simulink model "Jumper_Elastica"  (R2017b)
settings: Solver=ode15s  StartTime=0.0  StopTime=2  MaxStep=1e-2  RelTol=1e-3  EnableMultiTasking=on
InitFcn:
  | Variable_initialisation
values from neighbouring files (symbols this model uses):
  ArmatureResistance = 3.89    [Variable_initialisation.m]    (also in Variable_initialisation_shortleg.m; Variable_inizializzazione.m)
  ArmLength = 1.5    [Variable_initialisation.m]    (also in Variable_initialisation_shortleg.m; Variable_inizializzazione.m)
  ArmWidth = 0.1    [Variable_initialisation.m]    (also in Variable_initialisation_shortleg.m; Variable_inizializzazione.m)
  BaseX = Base*cos(BaseAngle)    [Variable_initialisation.m]    (also in Variable_initialisation_shortleg.m; Variable_inizializzazione.m; fourbar_initialisation.m)
  BaseY = Base*sin(BaseAngle)    [Variable_initialisation.m]    (also in Variable_initialisation_shortleg.m; Variable_inizializzazione.m; fourbar_initialisation.m)
  BodyMass = 1.0    (= 1)    [Variable_initialisation.m]    (also in Variable_initialisation_shortleg.m; Variable_inizializzazione.m = 1.4)
  FrontThigh = 30*Scale    (= 60)    [Variable_initialisation.m]    (also in Variable_initialisation_shortleg.m; Variable_inizializzazione.m; fourbar_initialisation.m = 45)
  GearRatio = 30    [Variable_initialisation.m]    (also in Variable_initialisation_shortleg.m; Variable_inizializzazione.m)
  Gravity = 9.81    [Variable_initialisation.m]    (also in Variable_initialisation_shortleg.m; Variable_inizializzazione.m)
  HardStop = 170    [Variable_initialisation.m]    (also in Variable_initialisation_shortleg.m; Variable_inizializzazione.m)
  InitialAngle = -113    [Variable_initialisation.m]    (also in Variable_initialisation_shortleg.m; Variable_inizializzazione.m)
  JumpingLegAttachPoint = -0.05    [Variable_initialisation.m]    (also in Variable_initialisation_shortleg.m = 0.05; Variable_inizializzazione.m)
  JumpingLegLength = 1.2    [Variable_initialisation.m]    (also in Variable_initialisation_shortleg.m = 0.9; Variable_inizializzazione.m = 0.8)
  JumpingLegMass = 0.3    [Variable_initialisation.m]    (also in Variable_initialisation_shortleg.m; Variable_inizializzazione.m = 0.5)
  JumpingLegStartAngle = rad2deg(asin(LandingLegHeight/JumpingLegCompressedLength))    [Variable_initialisation.m]    (also in Variable_initialisation_shortleg.m; Variable_inizializzazione.m)
  Knee = 5*Scale    (= 10)    [Variable_initialisation.m]    (also in Variable_initialisation_shortleg.m; Variable_inizializzazione.m; fourbar_initialisation.m)
  LandingLegHeight = 0.5    [Variable_initialisation.m]    (also in Variable_initialisation_shortleg.m; Variable_inizializzazione.m)
  LandingLegMass = 0.1    [Variable_initialisation.m]    (also in Variable_initialisation_shortleg.m; Variable_inizializzazione.m)
  MotorFreeSpeed = 2027    [Variable_initialisation.m]    (also in Variable_initialisation_shortleg.m; Variable_inizializzazione.m)
  MotorStallTorque = 2.32    [Variable_initialisation.m]    (also in Variable_initialisation_shortleg.m; Variable_inizializzazione.m)
  MotorVoltage = 16    [Variable_initialisation.m]    (also in Variable_initialisation_shortleg.m; Variable_inizializzazione.m)
  RearThigh = 29.5*Scale    (= 59)    [Variable_initialisation.m]    (also in Variable_initialisation_shortleg.m; Variable_inizializzazione.m; fourbar_initialisation.m = 43.5)
  SEA_Spring = 1e6    (= 1000000)    [Variable_initialisation.m]    (also in Variable_initialisation_shortleg.m; Variable_inizializzazione.m)
  Shin = 30*Scale    (= 60)    [Variable_initialisation.m]    (also in Variable_initialisation_shortleg.m; Variable_inizializzazione.m; fourbar_initialisation.m = 45)
undefined symbols (not defined in the file or in its folder): Beam, beam_wall, beam_width, Extr_Data_Box, magnitude, X, Y, Z
libraries: sm_lib x67, nesl_utility x25, fl_lib x21, simulink x8, Contact_Forces_Lib x7, sm_flex_body_lib x5, powerlib_meascontrol x2, mblibv1 x1, elec_lib x1
(part 1 of 3)
settings Model: Creator=rjs08  LastModifiedBy=rjs08
settings DataIOCC: LimitDataPoints=on
settings OptimizationCC: LifeSpan=inf
settings DebuggingCC: AllowSymbolicDim=off  SFUnexpectedBacktrackingDiag=warning  SFNoUnconditionalDefaultTransitionDiag=warning  SFExecutionAtInitializationDiag=none
settings CodeAppCC: StateflowObjectComments=on
settings GRTTargetCC: TargetLangStandard=C89/C90 (ANSI)  GeneratePreprocessorConditionals=Disable all
settings ConfigComp: CovMetricSettings=dw  CovHtmlReporting=on  CovSaveCumulativeToWorkspaceVar=on  CovSaveSingleToWorkspaceVar=on  CovExternalEMLEnable=off  CovSFcnEnable=off
settings SimscapeCC: SimscapeNominalValues="[{\"value\":\"10\",\"unit\":\"V\"},{\"value\":\"1\",\"unit\":\"A\"},{\"value\":\"10\",\"unit\":\"N*m\"},{\"value\":\"10\",\"unit\":\"bar\"},{\"value\":\"100\",\"unit\":\"kJ/kg\"},{\"value\":\"1\",\"unit\":\"kW\"},{\"value\":\"300\",\"unit\":\"K\"},{\"value\":\"100\",\"unit\":\"cm^3/s\"},{\"value\":\"1\",\"unit\":\"kN\"},{\"value\":\"1\",\"unit\":\"g/cm^3\"},{\"value\":\"1\",\"unit\":\"l\"},{\"value\":\"1\",\"unit\":\"cm^2\"},{\"value\":\"60\",\"unit\":\"Hz\"}]"  SimscapeLogType=all  SimscapeLogDataHistory=10000
settings ConfigurationSet: Description=SimMechanics 2G
settings DiagnosticsConfigSet: SimMechanicsRigidlyBoundBlock=none

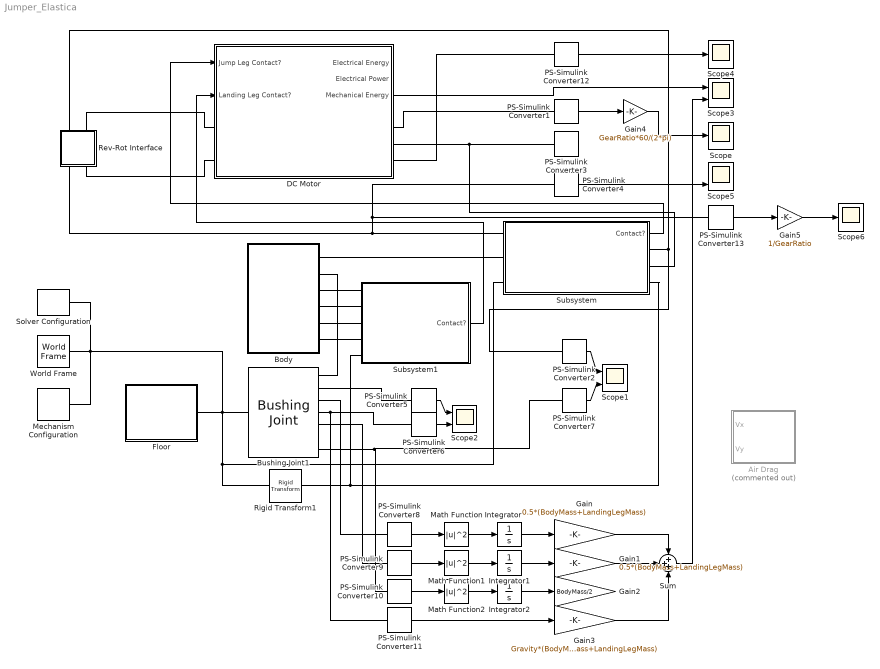
== system Jumper_Elastica ==
  Air Drag : Subsystem  Commented=on  mask(Air friction model){Cd=0}
      mask prompts: Cd "Drag Coefficient"
      mask help: Models aerodynamic drag. The drag coefficient Cd is a mask block parameter. Cd = 0 corresponds to zero drag. Cd = 2 corresponds to a sphere.
      mask init:
      | 0;
      mask Help: Enter aerodynamic drag coefficient Cd.  The block generates a three-vector of air friction as a function of 2D input velocity.
  Body : Subsystem  mask{L=ArmLength, L3=JumpingLegAttachPoint, W=ArmWidth, H=ArmWidth/2, M=BodyMass, LegH=LandingLegHeight, LegM=LandingLegMass, LegL=LandingLegHeight, rgb=[0 0 0]}
      mask prompts: L "Arm Length (m)"; L3 "Motor Mount Point (m)"; W "Arm Width (m)"; H "Body Thickness (m)"; M "Body Mass (kg)"; LegH "Leg Height (m)"; LegM "Leg Mass (kg)"; LegL "Leg Foot Length"; rgb "Color [R G B]"
  Bushing Joint1 : sm_lib/Joints/Bushing Joint  SenseConstraintForce=off  SenseConstraintForceX=off  SenseConstraintForceY=off  SenseConstraintForceZ=off  SenseConstraintTorque=off  SenseConstraintTorqueX=off  SenseConstraintTorqueY=off  SenseConstraintTorqueZ=off  SenseTotalForce=off  SenseTotalForceX=off  SenseTotalForceY=off  SenseTotalForceZ=off  SenseTotalTorque=off  SenseTotalTorqueX=off  SenseTotalTorqueY=off  SenseTotalTorqueZ=off  CompositeWrenchDir=FollowerOnBase  CompositeWrenchFrame=BaseFrame  PxEquilibriumPosition=0  PxEquilibriumPositionUnits=m  PxSpringStiffness=0  PxSpringStiffnessUnits=N/m  PxDampingCoefficient=0  PxDampingCoefficientUnits=N/(m/s)  PxTorqueActuationMode=NoTorque  PxMotionActuationMode=ComputedMotion  PxSensePosition=on  PxSenseVelocity=on  PxSenseAcceleration=off  PxSenseTorqueForce=off  PxPositionTargetSpecify=on  PxPositionTargetPriority=High  PxPositionTargetValue=0  PxPositionTargetValueUnits=m  PxVelocityTargetSpecify=off  PxVelocityTargetPriority=High  PxVelocityTargetValue=0  PxVelocityTargetValueUnits=m/s  PyEquilibriumPosition=0  PyEquilibriumPositionUnits=m  PySpringStiffness=0  PySpringStiffnessUnits=N/m  PyDampingCoefficient=0  PyDampingCoefficientUnits=N/(m/s)  PyTorqueActuationMode=NoTorque  PyMotionActuationMode=ComputedMotion  PySensePosition=on  PySenseVelocity=on  PySenseAcceleration=off  PySenseTorqueForce=off  PyPositionTargetSpecify=on  PyPositionTargetPriority=High  PyPositionTargetValue=0.05  PyPositionTargetValueUnits=m  PyVelocityTargetSpecify=off  PyVelocityTargetPriority=High  PyVelocityTargetValue=0  PyVelocityTargetValueUnits=m/s  PzEquilibriumPosition=0  PzEquilibriumPositionUnits=m  PzSpringStiffness=0  PzSpringStiffnessUnits=N/m  PzDampingCoefficient=0  PzDampingCoefficientUnits=N/(m/s)  PzTorqueActuationMode=NoTorque  PzMotionActuationMode=ComputedMotion  PzSensePosition=off  PzSenseVelocity=off  PzSenseAcceleration=off  PzSenseTorqueForce=off  PzPositionTargetSpecify=on  PzPositionTargetPriority=High  PzPositionTargetValue=0  PzPositionTargetValueUnits=m  PzVelocityTargetSpecify=off  PzVelocityTargetPriority=High  PzVelocityTargetValue=0  PzVelocityTargetValueUnits=m/s  RxEquilibriumPosition=0  RxEquilibriumPositionUnits=deg  RxSpringStiffness=0  RxSpringStiffnessUnits=N*m/deg  RxDampingCoefficient=0  RxDampingCoefficientUnits=N*m/(deg/s)  RxTorqueActuationMode=NoTorque  RxMotionActuationMode=ComputedMotion  RxSensePosition=off  RxSenseVelocity=off  RxSenseAcceleration=off  RxSenseTorqueForce=off  RxPositionTargetSpecify=on  RxPositionTargetPriority=High  RxPositionTargetValue=0  RxPositionTargetValueUnits=deg  RxVelocityTargetSpecify=off  RxVelocityTargetPriority=High  RxVelocityTargetValue=0  RxVelocityTargetValueUnits=deg/s  RyEquilibriumPosition=0  RyEquilibriumPositionUnits=deg  RySpringStiffness=0  RySpringStiffnessUnits=N*m/deg  RyDampingCoefficient=0  RyDampingCoefficientUnits=N*m/(deg/s)  RyTorqueActuationMode=NoTorque  RyMotionActuationMode=ComputedMotion  RySensePosition=off  RySenseVelocity=off  RySenseAcceleration=off  RySenseTorqueForce=off  RyPositionTargetSpecify=on  RyPositionTargetPriority=High  RyPositionTargetValue=0  RyPositionTargetValueUnits=deg  RyVelocityTargetSpecify=off  RyVelocityTargetPriority=High  RyVelocityTargetValue=0  RyVelocityTargetValueUnits=deg/s  RzEquilibriumPosition=0  RzEquilibriumPositionUnits=deg  RzSpringStiffness=0  RzSpringStiffnessUnits=N*m/deg  RzDampingCoefficient=0  RzDampingCoefficientUnits=N*m/(deg/s)  RzTorqueActuationMode=NoTorque  RzMotionActuationMode=ComputedMotion  RzSensePosition=on  RzSenseVelocity=on  RzSenseAcceleration=off  RzSenseTorqueForce=off  RzPositionTargetSpecify=on  RzPositionTargetPriority=High  RzPositionTargetValue=0  RzPositionTargetValueUnits=deg  RzVelocityTargetSpecify=off  RzVelocityTargetPriority=High  RzVelocityTargetValue=0  RzVelocityTargetValueUnits=deg/s
      settings: SourceProductName=Simscape Multibody
  DC Motor : Subsystem  mask{Stall_Torque=MotorStallTorque, Free_Speed=MotorFreeSpeed, Armature_Resistance=ArmatureResistance, Reverse_Point=0.3, Gear_Ratio=GearRatio, Motor_Voltage=MotorVoltage, SEA_Spring=SEA_Spring}
      mask prompts: Stall_Torque "Motor Stall Torque (Nm)"; Free_Speed "Motor Free Speed (rpm)"; Armature_Resistance "Motor Armature Resistance (ohm)"; Reverse_Point "Reverse Point (ignore)"; Gear_Ratio "Gear Reduction Ratio"; Motor_Voltage "Motor Voltage (V)"; SEA_Spring "SEA Spring (Nm/rad)"
  Floor : Subsystem  mask{L=2, W=2, H=0.01, M=2}
      mask prompts: L "Length (m)"; W "Width (m)"; H "Height (m)"; M "Mass (kg)"
  Gain : Gain  Gain=0.5*(BodyMass+LandingLegMass)
  Gain1 : Gain  Gain=0.5*(BodyMass+LandingLegMass)
  Gain2 : Gain  Gain=BodyMass/2
  Gain3 : Gain  Gain=Gravity*(BodyMass+LandingLegMass)
  Gain4 : Gain  Gain=GearRatio*60/(2*pi)
  Gain5 : Gain  Gain=1/GearRatio
  Integrator : Integrator
  Integrator1 : Integrator
  Integrator2 : Integrator
  Math Function : Math  Operator=magnitude^2  SaturateOnIntegerOverflow=on
  Math Function1 : Math  Operator=magnitude^2  SaturateOnIntegerOverflow=on
  Math Function2 : Math  Operator=magnitude^2  SaturateOnIntegerOverflow=on
  Mechanism Configuration : sm_lib/Utilities/Mechanism Configuration  UniformGravity=Constant  GravityVector=[0 -Gravity 0]  GravityUnits=m/s^2  LinearizationDelta=0.001
  PS-Simulink Converter{1..13} (13 alike) : nesl_utility/PS-Simulink Converter  PhysicalDomain=network_engine_domain  SubClassName=ps_output  LeftPortType=input  RightPortType=output  PseudoPeriodic=off  Frequencies=[]  Unit=1  AffineConversion=off
  Rev-Rot Interface : Subsystem
  Rigid Transform1 : sm_lib/Frames and Transforms/Rigid Transform  TranslationMethod=StandardAxis  TranslationStandardOffset=3  TranslationLengthUnit=m  TranslationStandardAxis=+X  TranslationCartesianOffset=[0 0 0]  TranslationROffset=0  TranslationROffsetUnits=m  TranslationZOffset=0  TranslationZOffsetUnits=m  TranslationThetaOffset=0  TranslationThetaOffsetUnits=deg  RotationMethod=StandardAxis  RotationAngleUnits=deg  RotationStandardAxis=+X  RotationAngle=90  RotationArbitraryAxis=[0 0 1]  FollAlignAxisA=+X  BaseAlignAxisA=+Y  FollAlignAxisB=+Y  BaseAlignAxisB=+Z  RotationSequenceAxes=FollowerAxes  RotationSequence=XYX  RotationSequenceAngles=[0 0 0]  RotationSequenceAnglesUnits=deg  RotationMatrix=[1 0 0; 0 1 0; 0 0 1]
  Scope : Scope
  Scope1 : Scope  NumInputPorts=2
  Scope2 : Scope  NumInputPorts=2
  Scope3 : Scope  NumInputPorts=2
  Scope4 : Scope
  Scope5 : Scope  NumInputPorts=3
  Scope6 : Scope
  Solver Configuration : nesl_utility/Solver Configuration  PhysicalDomain=network_engine_domain  SubClassName=solver  LeftPortType=input  RightPortType=generic  Accelerate=off  Tones=[]  Harmonics=[]  SimulateNoise=off  Profile=off  UseLocalSampling=off  EnableSwitchedLinearOptims=on  FrequencyDomain=off  UseCCode=off  RelTol=0.001  AbsTol=1e-06  MinStep=1e-09  ToWorkspace=off  RevertToSquareIcSolve=off  NumHomotopyIterations=100  PhasorMode=off  PhasorModeNumHarmonics=1  DoDC=off  ResidualTolerance=1e-09  UseLocalSolver=off  LocalSolverChoice=NE_BACKWARD_EULER_ADVANCER  LocalSolverSampleTime=0.001  DoFixedCost=off  MaxNonlinIter=3  MaxModeIter=2  LinearAlgebra=Sparse  DelaysMemoryBudget=1024  AutomaticFiltering=on  FilteringTimeConstant=0.001
  Subsystem : Subsystem
  Subsystem1 : Subsystem
  Sum : Sum  Inputs=+++
  World Frame : sm_lib/Frames and Transforms/World Frame
  wires:
  PS-Simulink Converter1/1 -> Gain4/1
  PS-Simulink Converter6/1 -> Scope2/2
  PS-Simulink Converter5/1 -> Scope2/1
  Subsystem/1(Contact?) -> DC Motor/1(Jump Leg Contact?)
  Subsystem1/1(Contact?) -> DC Motor/2(Landing Leg Contact?)
  PS-Simulink Converter2/1 -> Scope1/1
  PS-Simulink Converter7/1 -> Scope1/2
  DC Motor/3(Mechanical Energy) -> Scope3/1
  PS-Simulink Converter8/1 -> Math Function/1
  PS-Simulink Converter9/1 -> Math Function1/1
  PS-Simulink Converter10/1 -> Math Function2/1
  Integrator/1 -> Gain/1
  Integrator1/1 -> Gain1/1
  PS-Simulink Converter11/1 -> Gain3/1
  Integrator2/1 -> Gain2/1
  Math Function/1 -> Integrator/1
  Math Function1/1 -> Integrator1/1
  Math Function2/1 -> Integrator2/1
  Gain1/1 -> Sum/2
  Gain/1 -> Sum/1
  Gain3/1 -> Sum/3
  Sum/1 -> Scope3/2
  PS-Simulink Converter4/1 -> Scope5/3
  Gain4/1 -> Scope/1
  PS-Simulink Converter13/1 -> Gain5/1
  Gain5/1 -> Scope6/1
  PS-Simulink Converter12/1 -> Scope4/1
  connections:
  Body/RConn2 -- Bushing Joint1/RConn1
  Bushing Joint1/LConn1 -- Solver Configuration/RConn1 -- Mechanism Configuration/RConn1 -- World Frame/RConn1 -- Rigid Transform1/LConn1 -- Subsystem/LConn3 -- Floor/RConn1
  DC Motor/LConn2 -- Rev-Rot Interface/LConn2
  DC Motor/LConn1 -- Rev-Rot Interface/RConn2
  PS-Simulink Converter1/LConn1 -- DC Motor/RConn2
  DC Motor/RConn3 -- Subsystem/RConn2 -- PS-Simulink Converter3/LConn1
  Rev-Rot Interface/LConn1 -- PS-Simulink Converter13/LConn1 -- PS-Simulink Converter4/LConn1 -- Subsystem/LConn1
  Rev-Rot Interface/RConn1 -- Subsystem/RConn1 -- PS-Simulink Converter2/LConn1
  Subsystem/LConn2 -- Body/RConn1
  Subsystem/RConn3 -- Subsystem1/LConn5 -- Rigid Transform1/RConn1
  Body/RConn3 -- Subsystem1/LConn1
  Subsystem1/LConn2 -- Body/RConn4
  Subsystem1/LConn3 -- Body/RConn5
  Subsystem1/LConn4 -- Body/RConn6
  PS-Simulink Converter6/LConn1 -- PS-Simulink Converter11/LConn1 -- Bushing Joint1/RConn4
  Bushing Joint1/RConn3 -- PS-Simulink Converter8/LConn1
  PS-Simulink Converter9/LConn1 -- Bushing Joint1/RConn5
  Bushing Joint1/RConn7 -- PS-Simulink Converter7/LConn1 -- PS-Simulink Converter10/LConn1
  PS-Simulink Converter12/LConn1 -- DC Motor/RConn4
  PS-Simulink Converter5/LConn1 -- Bushing Joint1/RConn2

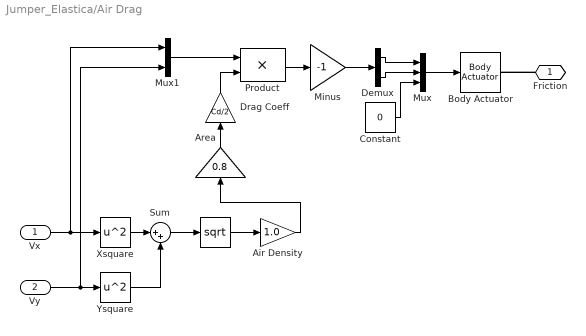
== system Jumper_Elastica/Air Drag ==
  Vx : Inport
  Vy : Inport  Port=2
  " " : Math  Operator=sqrt  SaturateOnIntegerOverflow=on
  Air Density : Gain  Gain=1.0  SaturateOnIntegerOverflow=on  OutDataTypeStr=Inherit: Same as input  ParamDataTypeStr=Inherit: Same as input
  Area : Gain  Gain=0.8  SaturateOnIntegerOverflow=on  OutDataTypeStr=Inherit: Same as input  ParamDataTypeStr=Inherit: Same as input
  Body Actuator : mblibv1/Sensors &  Actuators/Body Actuator  UpdateFromCAD=off  PhysicalDomain=Mechanical  PortType=blob  ActuationStyle=Force  AngleUnits=deg  ArcVelocityUnits=deg/s  ArcAccelerationUnits=deg/s^2  CoordPositionUnits=m  VelocityUnits=m/s  AccelerationUnits=m/s^2  ForceUnits=N  TorqueUnits=N-m  ActiveIO=off  Width=3  DialogClass=MechanicalActuatorBlock  ReferenceFrame=Absolute (World)  Angle=off  CoordPosition=on  Force=on  Torque=off
      settings: SourceProductName=Simscape Multibody  SourceProductBaseCode=MS
  Constant : Constant  Value=0
  Demux : Demux  Outputs=2
  Drag Coeff : Gain  Gain=Cd/2  SaturateOnIntegerOverflow=on  OutDataTypeStr=Inherit: Same as input  ParamDataTypeStr=Inherit: Same as input
  Minus : Gain  Gain=-1  SaturateOnIntegerOverflow=on  OutDataTypeStr=Inherit: Same as input  ParamDataTypeStr=Inherit: Same as input
  Mux : Mux  Inputs=3
  Mux1 : Mux  Inputs=2
  Product : Product  SaturateOnIntegerOverflow=on  OutDataTypeStr=Inherit: Same as first input
  Sum : Sum  Inputs=|++  SaturateOnIntegerOverflow=on
  Xsquare : Math  Operator=square  SaturateOnIntegerOverflow=on
  Ysquare : Math  Operator=square  SaturateOnIntegerOverflow=on
  Friction : PMIOPort  Port=1  Side=Right
  wires:
  Vx/1 -> Mux1/1, Xsquare/1
  Xsquare/1 -> Sum/1
  Ysquare/1 -> Sum/2
  Mux/1 -> Body Actuator/1
  Constant/1 -> Mux/3
  Area/1 -> Drag Coeff/1
  Mux1/1 -> Product/1
  Vy/1 -> Mux1/2, Ysquare/1
  Drag Coeff/1 -> Product/2
  Air Density/1 -> Area/1
  Sum/1 -> " "/1
  " "/1 -> Air Density/1
  Product/1 -> Minus/1
  Minus/1 -> Demux/1
  Demux/2 -> Mux/2
  Demux/1 -> Mux/1
  connections:
  Friction/RConn1 -- Body Actuator/RConn1

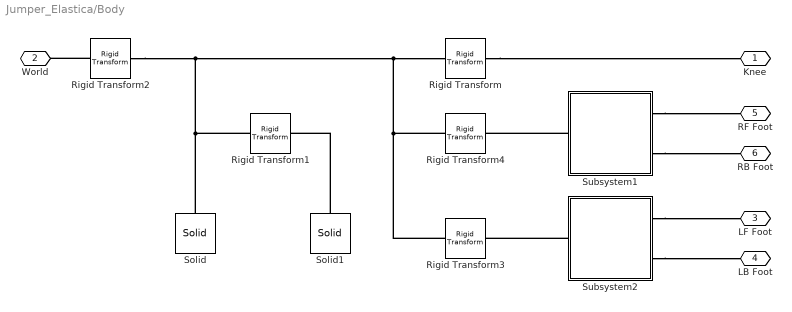
== system Jumper_Elastica/Body ==
  Rigid Transform : sm_lib/Frames and Transforms/Rigid Transform  TranslationMethod=StandardAxis  TranslationStandardOffset=L3  TranslationLengthUnit=m  TranslationStandardAxis=-X  TranslationCartesianOffset=[0 0 0]  TranslationROffset=0  TranslationROffsetUnits=m  TranslationZOffset=0  TranslationZOffsetUnits=m  TranslationThetaOffset=0  TranslationThetaOffsetUnits=deg  RotationMethod=None  RotationAngleUnits=deg  RotationStandardAxis=+Z  RotationAngle=0.0  RotationArbitraryAxis=[0 0 1]  FollAlignAxisA=+X  BaseAlignAxisA=+Y  FollAlignAxisB=+Y  BaseAlignAxisB=+Z  RotationSequenceAxes=FollowerAxes  RotationSequence=XYX  RotationSequenceAngles=[0 0 0]  RotationSequenceAnglesUnits=deg  RotationMatrix=[1 0 0; 0 1 0; 0 0 1]
  Rigid Transform1 : sm_lib/Frames and Transforms/Rigid Transform  TranslationMethod=None  TranslationStandardOffset=L/2  TranslationLengthUnit=m  TranslationStandardAxis=-X  TranslationCartesianOffset=[0 0 0]  TranslationROffset=0  TranslationROffsetUnits=m  TranslationZOffset=0  TranslationZOffsetUnits=m  TranslationThetaOffset=0  TranslationThetaOffsetUnits=deg  RotationMethod=StandardAxis  RotationAngleUnits=deg  RotationStandardAxis=+Y  RotationAngle=90  RotationArbitraryAxis=[0 0 1]  FollAlignAxisA=+X  BaseAlignAxisA=+Y  FollAlignAxisB=+Y  BaseAlignAxisB=+Z  RotationSequenceAxes=FollowerAxes  RotationSequence=XYX  RotationSequenceAngles=[0 0 0]  RotationSequenceAnglesUnits=deg  RotationMatrix=[1 0 0; 0 1 0; 0 0 1]
  Rigid Transform2 : sm_lib/Frames and Transforms/Rigid Transform  TranslationMethod=StandardAxis  TranslationStandardOffset=LegH  TranslationLengthUnit=m  TranslationStandardAxis=+Y  TranslationCartesianOffset=[0 0 0]  TranslationROffset=0  TranslationROffsetUnits=m  TranslationZOffset=0  TranslationZOffsetUnits=m  TranslationThetaOffset=0  TranslationThetaOffsetUnits=deg  RotationMethod=None  RotationAngleUnits=deg  RotationStandardAxis=+Z  RotationAngle=0.0  RotationArbitraryAxis=[0 0 1]  FollAlignAxisA=+X  BaseAlignAxisA=+Y  FollAlignAxisB=+Y  BaseAlignAxisB=+Z  RotationSequenceAxes=FollowerAxes  RotationSequence=XYX  RotationSequenceAngles=[0 0 0]  RotationSequenceAnglesUnits=deg  RotationMatrix=[1 0 0; 0 1 0; 0 0 1]
  Rigid Transform3 : sm_lib/Frames and Transforms/Rigid Transform  TranslationMethod=StandardAxis  TranslationStandardOffset=L/4  TranslationLengthUnit=m  TranslationStandardAxis=-Z  TranslationCartesianOffset=[0 0 0]  TranslationROffset=0  TranslationROffsetUnits=m  TranslationZOffset=0  TranslationZOffsetUnits=m  TranslationThetaOffset=0  TranslationThetaOffsetUnits=deg  RotationMethod=None  RotationAngleUnits=deg  RotationStandardAxis=+Z  RotationAngle=0.0  RotationArbitraryAxis=[0 0 1]  FollAlignAxisA=+X  BaseAlignAxisA=+Y  FollAlignAxisB=+Y  BaseAlignAxisB=+Z  RotationSequenceAxes=FollowerAxes  RotationSequence=XYX  RotationSequenceAngles=[0 0 0]  RotationSequenceAnglesUnits=deg  RotationMatrix=[1 0 0; 0 1 0; 0 0 1]
  Rigid Transform4 : sm_lib/Frames and Transforms/Rigid Transform  TranslationMethod=StandardAxis  TranslationStandardOffset=L/4  TranslationLengthUnit=m  TranslationStandardAxis=+Z  TranslationCartesianOffset=[0 0 0]  TranslationROffset=0  TranslationROffsetUnits=m  TranslationZOffset=0  TranslationZOffsetUnits=m  TranslationThetaOffset=0  TranslationThetaOffsetUnits=deg  RotationMethod=None  RotationAngleUnits=deg  RotationStandardAxis=+Z  RotationAngle=0.0  RotationArbitraryAxis=[0 0 1]  FollAlignAxisA=+X  BaseAlignAxisA=+Y  FollAlignAxisB=+Y  BaseAlignAxisB=+Z  RotationSequenceAxes=FollowerAxes  RotationSequence=XYX  RotationSequenceAngles=[0 0 0]  RotationSequenceAnglesUnits=deg  RotationMatrix=[1 0 0; 0 1 0; 0 0 1]
  Solid : sm_lib/Body Elements/Solid  InertiaType=CalculateFromGeometry  Mass=M/2  MassUnits=kg  CenterOfMass=[0 0 0]  CenterOfMassUnits=m  MomentsOfInertia=[1 1 1]  MomentsOfInertiaUnits=kg*m^2  ProductsOfInertia=[1 1 1]  ProductsOfInertiaUnits=kg*m^2  DensityBased=off  Density=1000  DensityUnits=kg/m^3  DoExposeReferenceFrame=on  SerializedFrames=<Frames/>  GraphicType=FromGeometry  MarkerShape=Sphere  MarkerSize=10  GraphicVisPropType=SimpleVisualProperties  GraphicDiffuseColor=rgb  GraphicSpecularColor=[0.5 0.5 0.5 1.0]  GraphicAmbientColor=[0.15 0.15 0.15 1.0]  GraphicEmissiveColor=[0.0 0.0 0.0 1.0]  GraphicShininess=75  GraphicOpacity=0.5  GeometryShape=Brick  RectangleSize=[1 1]  RectangleSizeUnits=m  BrickDimensions=[L H W]  BrickDimensionUnits=m  CylinderRadius=1  CylinderRadiusUnits=m  CylinderLength=1  CylinderLengthUnits=m  SphereRadius=1  SphereRadiusUnits=m  EllipsoidRadii=[1 1 1]  EllipsoidRadiiUnits=m  ExtrusionCrossSection=[1 1; -1 1; -1 -1; 1 -1]  ExtrusionCrossSectionUnits=m  ExtrusionLength=1  ExtrusionLengthUnits=m  PolygonNumSides=3  PolygonOuterRadius=1  PolygonOuterRadiusUnits=m  ExtGeomFileType=STEP  ExtGeomFileUnits=m  RevolutionCrossSection=[1 1; 1 -1; 2 -1; 2 1]  RevolutionCrossSectionUnits=m  RevolutionExtent=Full  RevolutionAngle=180  RevolutionAngleUnits=deg
  Solid1 : sm_lib/Body Elements/Solid  InertiaType=CalculateFromGeometry  Mass=M/2  MassUnits=kg  CenterOfMass=[0 0 0]  CenterOfMassUnits=m  MomentsOfInertia=[1 1 1]  MomentsOfInertiaUnits=kg*m^2  ProductsOfInertia=[1 1 1]  ProductsOfInertiaUnits=kg*m^2  DensityBased=off  Density=1000  DensityUnits=kg/m^3  DoExposeReferenceFrame=on  SerializedFrames=<Frames/>  GraphicType=FromGeometry  MarkerShape=Sphere  MarkerSize=10  GraphicVisPropType=SimpleVisualProperties  GraphicDiffuseColor=rgb  GraphicSpecularColor=[0.5 0.5 0.5 1.0]  GraphicAmbientColor=[0.15 0.15 0.15 1.0]  GraphicEmissiveColor=[0.0 0.0 0.0 1.0]  GraphicShininess=75  GraphicOpacity=0.5  GeometryShape=Brick  RectangleSize=[1 1]  RectangleSizeUnits=m  BrickDimensions=[L H W]  BrickDimensionUnits=m  CylinderRadius=1  CylinderRadiusUnits=m  CylinderLength=1  CylinderLengthUnits=m  SphereRadius=1  SphereRadiusUnits=m  EllipsoidRadii=[1 1 1]  EllipsoidRadiiUnits=m  ExtrusionCrossSection=[1 1; -1 1; -1 -1; 1 -1]  ExtrusionCrossSectionUnits=m  ExtrusionLength=1  ExtrusionLengthUnits=m  PolygonNumSides=3  PolygonOuterRadius=1  PolygonOuterRadiusUnits=m  ExtGeomFileType=STEP  ExtGeomFileUnits=m  RevolutionCrossSection=[1 1; 1 -1; 2 -1; 2 1]  RevolutionCrossSectionUnits=m  RevolutionExtent=Full  RevolutionAngle=180  RevolutionAngleUnits=deg
  Subsystem1 : Subsystem
  Subsystem2 : Subsystem
  Knee : PMIOPort  Port=1  Side=Right
  World : PMIOPort  Port=2  Side=Right
  LF Foot : PMIOPort  Port=3  Side=Right
  " LB Foot" : PMIOPort  Port=4  Side=Right
  RF Foot : PMIOPort  Port=5  Side=Right
  " RB Foot" : PMIOPort  Port=6  Side=Right
  connections:
  Rigid Transform/RConn1 -- Knee/RConn1
  Solid1/RConn1 -- Rigid Transform1/RConn1
  Rigid Transform2/LConn1 -- World/RConn1
  Rigid Transform2/RConn1 -- Rigid Transform1/LConn1 -- Solid/RConn1 -- Rigid Transform4/LConn1 -- Rigid Transform3/LConn1 -- Rigid Transform/LConn1
  Subsystem2/RConn2 -- " LB Foot"/RConn1
  Subsystem2/RConn1 -- LF Foot/RConn1
  Subsystem2/LConn1 -- Rigid Transform3/RConn1
  Subsystem1/RConn1 -- RF Foot/RConn1
  Subsystem1/RConn2 -- " RB Foot"/RConn1
  Subsystem1/LConn1 -- Rigid Transform4/RConn1

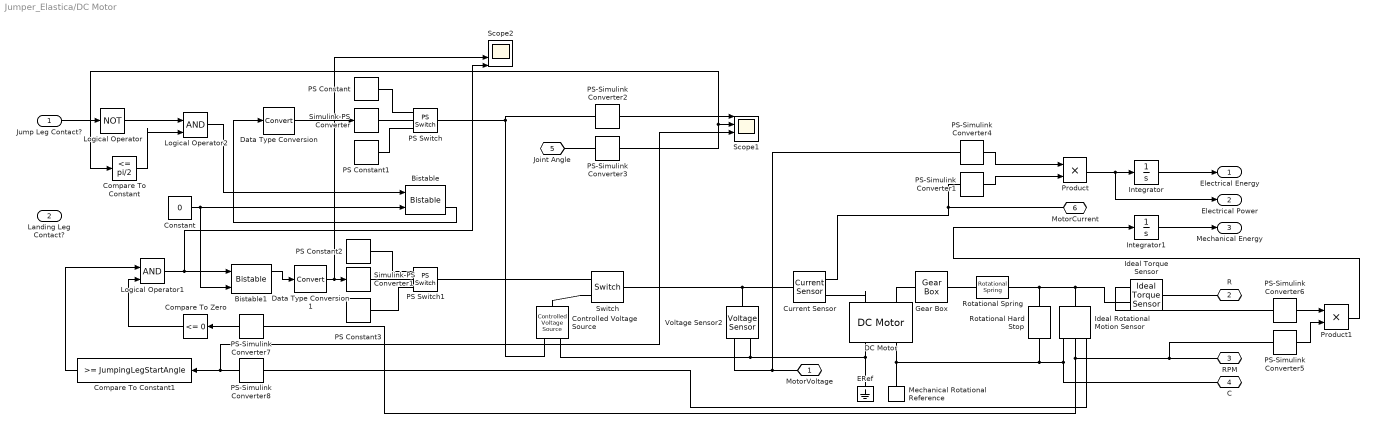
== system Jumper_Elastica/DC Motor ==
  Jump Leg Contact? : Inport
  Landing Leg Contact? : Inport  Port=2
  Bistable : powerlib_meascontrol/Logic/Bistable  Qpriority=Set  ic=0  Ts=0
      settings: SourceProductName=Simscape Power Systems  SourceProductBaseCode=PS
  Bistable1 : powerlib_meascontrol/Logic/Bistable  Qpriority=Set  ic=0  Ts=0
      settings: SourceProductName=Simscape Power Systems  SourceProductBaseCode=PS
  Compare To Constant : simulink/Logic and Bit Operations/Compare To Constant  relop=<=  const=pi/2  OutDataTypeStr=boolean
  Compare To Constant1 : simulink/Logic and Bit Operations/Compare To Constant  relop=>=  const=JumpingLegStartAngle  OutDataTypeStr=boolean
  Compare To Zero : simulink/Logic and Bit Operations/Compare To Zero  relop=<=  OutDataTypeStr=boolean
  Constant : Constant  Value=0  OutDataTypeStr=boolean
  Controlled Voltage Source : fl_lib/Electrical/Electrical Sources/Controlled Voltage Source
  Current Sensor : fl_lib/Electrical/Electrical Sensors/Current Sensor
  DC Motor : elec_lib/Actuators & Drivers/Rotational Actuators/DC Motor  parameterization=2  Ra=3.9 Ohm  La=12e-9 H  emf_or_torque=1  Kv=0.072e-3 V/rpm  Ki=6.876e-4 N*m/A  T_stall=Stall_Torque N*m  w_max=Free_Speed rpm  w_rated=15000 rpm  P_rated=0.08 W  V_rated=12 V  J=0 g*cm^2  lam_param=2  lam=0 N*m/(rad/s)  i_noload=12/Armature_Resistance A  V_i_noload=12 V  speed0=0 rpm  alpha=3.93e-3 1/K  Tmeas=25 degC  thermal_mass=100 J/K  initial_temperature=25 degC
  Data Type Conversion : DataTypeConversion
  Data Type Conversion1 : DataTypeConversion
  ERef : fl_lib/Electrical/Electrical Elements/Electrical Reference
      settings: SourceProductName=Foundation Library
  Gear Box : fl_lib/Mechanical/Mechanisms/Gear Box  ratio=Gear_Ratio  t_in_specify=off  t_in_priority=None  t_in=0 N*m  t_in_nominal_specify=off  t_in_nominal_unit=N*m  t_in_nominal_value=1  t_out_specify=off  t_out_priority=None  t_out=0 N*m  t_out_nominal_specify=off  t_out_nominal_unit=N*m  t_out_nominal_value=1
  Ideal Rotational Motion Sensor : fl_lib/Mechanical/Mechanical Sensors/Ideal Rotational Motion Sensor  offset=0 rad
  Ideal Torque Sensor : fl_lib/Mechanical/Mechanical Sensors/Ideal Torque Sensor
  Integrator : Integrator
  Integrator1 : Integrator
  Logical Operator : Logic  Operator=NOT  IconShape=distinctive  AllPortsSameDT=off  OutDataTypeStr=boolean
  Logical Operator1 : Logic  IconShape=distinctive  AllPortsSameDT=off  OutDataTypeStr=boolean
  Logical Operator2 : Logic  IconShape=distinctive  AllPortsSameDT=off  OutDataTypeStr=boolean
  Mechanical Rotational Reference : fl_lib/Mechanical/Rotational Elements/Mechanical Rotational Reference
  PS Constant : fl_lib/Physical Signals/Sources/PS Constant  constant=-Motor_Voltage
  PS Constant1 : fl_lib/Physical Signals/Sources/PS Constant  constant=Motor_Voltage
  PS Constant2 : fl_lib/Physical Signals/Sources/PS Constant  constant=0
  PS Constant3 : fl_lib/Physical Signals/Sources/PS Constant  constant=2
  PS Switch : fl_lib/Physical Signals/Nonlinear Operators/PS Switch  Threshold=0.5
      settings: SourceProductName=Simscape  SourceProductBaseCode=SS
  PS Switch1 : fl_lib/Physical Signals/Nonlinear Operators/PS Switch  Threshold=0.5
      settings: SourceProductName=Simscape  SourceProductBaseCode=SS
  PS-Simulink Converter{1..8} (8 alike) : nesl_utility/PS-Simulink Converter  PhysicalDomain=network_engine_domain  SubClassName=ps_output  LeftPortType=input  RightPortType=output  PseudoPeriodic=off  Frequencies=[]  Unit=1  AffineConversion=off
  Product : Product
  Product1 : Product
  Rotational Hard Stop : fl_lib/Mechanical/Rotational Elements/Rotational Hard Stop  upper_bnd=JumpingLegStartAngle deg  lower_bnd=-HardStop+JumpingLegStartAngle deg  stiff_up=1e6 N*m/rad  stiff_low=1e6 N*m/rad  D_up=0.01 N*m/(rad/s)  D_low=0.01 N*m/(rad/s)  model=2  transition=0.001 rad  w_specify=off  w_priority=None  w=0 rad/s  w_nominal_specify=off  w_nominal_unit=rad/s  w_nominal_value=1  t_specify=off  t_priority=None  t=0 N*m  t_nominal_specify=off  t_nominal_unit=N*m  t_nominal_value=1  phi_specify=off  phi_priority=High  phi=0 rad  phi_nominal_specify=off  phi_nominal_unit=rad  phi_nominal_value=1
      settings: SourceProductName=Simscape  SourceProductBaseCode=SS
  Rotational Spring : fl_lib/Mechanical/Rotational Elements/Rotational Spring  spr_rate=SEA_Spring N*m/rad  w_specify=off  w_priority=None  w=0 rad/s  w_nominal_specify=off  w_nominal_unit=rad/s  w_nominal_value=1  t_specify=off  t_priority=None  t=0 N*m  t_nominal_specify=off  t_nominal_unit=N*m  t_nominal_value=1  phi_specify=off  phi_priority=High  phi=0 rad  phi_nominal_specify=off  phi_nominal_unit=rad  phi_nominal_value=1
      settings: SourceProductName=Simscape
  Scope1 : Scope  NumInputPorts=4
  Scope2 : Scope  NumInputPorts=4
  Simulink-PS Converter : nesl_utility/Simulink-PS Converter  PhysicalDomain=network_engine_domain  SubClassName=ps_input  LeftPortType=input  RightPortType=output  PseudoPeriodic=off  Frequencies=[]  NoiseDistribution=none  NoiseParameters=[]  Unit=1  AffineConversion=off  FilteringAndDerivatives=provide  SimscapeFilterOrder=1  InputFilterTimeConstant=0.001  UdotUserProvided=0
  Simulink-PS Converter1 : nesl_utility/Simulink-PS Converter  PhysicalDomain=network_engine_domain  SubClassName=ps_input  LeftPortType=input  RightPortType=output  PseudoPeriodic=off  Frequencies=[]  NoiseDistribution=none  NoiseParameters=[]  Unit=1  AffineConversion=off  FilteringAndDerivatives=provide  SimscapeFilterOrder=1  InputFilterTimeConstant=0.001  UdotUserProvided=0
  Switch : fl_lib/Electrical/Electrical Elements/Switch  R_closed=0.01 Ohm  G_open=1e-8 1/Ohm  Threshold=1  i_specify=off  i_priority=None  i=0 A  i_nominal_specify=off  i_nominal_unit=A  i_nominal_value=1  v_specify=off  v_priority=None  v=0 V  v_nominal_specify=off  v_nominal_unit=V  v_nominal_value=1
      settings: SourceProductName=Simscape
  Voltage Sensor2 : fl_lib/Electrical/Electrical Sensors/Voltage Sensor
  "MotorVoltage " : PMIOPort  Port=1  Side=Right
  R : PMIOPort  Port=2  Side=Left
  RPM : PMIOPort  Port=3  Side=Right
  C : PMIOPort  Port=4  Side=Left
  Joint Angle : PMIOPort  Port=5  Side=Right
  MotorCurrent : PMIOPort  Port=6  Side=Right
  Electrical Energy : Outport
  Electrical Power : Outport  Port=2
  Mechanical Energy : Outport  Port=3
  wires:
  PS-Simulink Converter2/1 -> Scope1/1
  PS-Simulink Converter3/1 -> Compare To Constant/1, Scope1/2
  PS-Simulink Converter4/1 -> Product/1
  PS-Simulink Converter1/1 -> Product/2
  Product/1 -> Electrical Power/1, Integrator/1
  Integrator/1 -> Electrical Energy/1
  Jump Leg Contact?/1 -> Logical Operator/1
  Constant/1 -> Bistable/2, Bistable1/2
  Logical Operator/1 -> Logical Operator2/1
  Data Type Conversion/1 -> Simulink-PS Converter/1
  Logical Operator2/1 -> Bistable/1
  Compare To Constant/1 -> Logical Operator2/2
  Bistable/2 -> Data Type Conversion/1
  Integrator1/1 -> Mechanical Energy/1
  PS-Simulink Converter6/1 -> Product1/1
  PS-Simulink Converter5/1 -> Product1/2
  Product1/1 -> Integrator1/1
  Bistable1/1 -> Data Type Conversion1/1
  Data Type Conversion1/1 -> Scope2/3, Simulink-PS Converter1/1
  Logical Operator1/1 -> Scope2/4, Bistable1/1
  PS-Simulink Converter7/1 -> Compare To Zero/1
  PS-Simulink Converter8/1 -> Compare To Constant1/1, Scope1/3
  Compare To Zero/1 -> Logical Operator1/2
  Compare To Constant1/1 -> Logical Operator1/1
  connections:
  RPM/RConn1 -- PS-Simulink Converter5/LConn1 -- PS-Simulink Converter7/LConn1 -- Ideal Rotational Motion Sensor/RConn2
  Mechanical Rotational Reference/LConn1 -- Rotational Hard Stop/RConn1 -- C/RConn1 -- Ideal Rotational Motion Sensor/RConn1 -- DC Motor/RConn2
  Voltage Sensor2/RConn1 -- PS-Simulink Converter4/LConn1 -- "MotorVoltage "/RConn1
  PS Switch/RConn1 -- Controlled Voltage Source/RConn1 -- PS-Simulink Converter2/LConn1
  PS Constant/RConn1 -- PS Switch/LConn1
  PS Constant1/RConn1 -- PS Switch/LConn3
  DC Motor/RConn1 -- Controlled Voltage Source/RConn2 -- Voltage Sensor2/RConn2 -- ERef/LConn1
  DC Motor/LConn1 -- Current Sensor/RConn2
  Current Sensor/RConn1 -- PS-Simulink Converter1/LConn1 -- MotorCurrent/RConn1
  Current Sensor/LConn1 -- Switch/LConn1 -- Voltage Sensor2/LConn1
  PS Constant2/RConn1 -- PS Switch1/LConn1
  PS Constant3/RConn1 -- PS Switch1/LConn3
  PS-Simulink Converter3/LConn1 -- Joint Angle/RConn1
  PS-Simulink Converter6/LConn1 -- Ideal Torque Sensor/RConn2
  R/RConn1 -- Ideal Torque Sensor/LConn1
  PS Switch1/LConn2 -- Simulink-PS Converter1/RConn1
  Ideal Rotational Motion Sensor/RConn3 -- PS-Simulink Converter8/LConn1
  Switch/RConn2 -- Controlled Voltage Source/LConn1
  Switch/RConn1 -- PS Switch1/RConn1
  DC Motor/LConn2 -- Gear Box/LConn1
  Rotational Spring/LConn1 -- Gear Box/RConn1
  Ideal Torque Sensor/RConn1 -- Ideal Rotational Motion Sensor/LConn1 -- Rotational Hard Stop/LConn1 -- Rotational Spring/RConn1
  PS Switch/LConn2 -- Simulink-PS Converter/RConn1

== system Jumper_Elastica/Floor ==
  Rigid Transform : sm_lib/Frames and Transforms/Rigid Transform  TranslationMethod=StandardAxis  TranslationStandardOffset=L/2  TranslationLengthUnit=m  TranslationStandardAxis=-X  TranslationCartesianOffset=[0 0 0]  TranslationROffset=0  TranslationROffsetUnits=m  TranslationZOffset=0  TranslationZOffsetUnits=m  TranslationThetaOffset=0  TranslationThetaOffsetUnits=deg  RotationMethod=None  RotationAngleUnits=deg  RotationStandardAxis=+Z  RotationAngle=0.0  RotationArbitraryAxis=[0 0 1]  FollAlignAxisA=+X  BaseAlignAxisA=+Y  FollAlignAxisB=+Y  BaseAlignAxisB=+Z  RotationSequenceAxes=FollowerAxes  RotationSequence=XYX  RotationSequenceAngles=[0 0 0]  RotationSequenceAnglesUnits=deg  RotationMatrix=[1 0 0; 0 1 0; 0 0 1]
  Solid : sm_lib/Body Elements/Solid  InertiaType=CalculateFromGeometry  Mass=M  MassUnits=kg  CenterOfMass=[0 0 0]  CenterOfMassUnits=m  MomentsOfInertia=[1 1 1]  MomentsOfInertiaUnits=kg*m^2  ProductsOfInertia=[1 1 1]  ProductsOfInertiaUnits=kg*m^2  DensityBased=off  Density=1000  DensityUnits=kg/m^3  DoExposeReferenceFrame=on  SerializedFrames=<Frames/>  GraphicType=FromGeometry  MarkerShape=Sphere  MarkerSize=10  GraphicVisPropType=SimpleVisualProperties  GraphicDiffuseColor=[0.8 0.45 0.]  GraphicSpecularColor=[0.5 0.5 0.5 1.0]  GraphicAmbientColor=[0.15 0.15 0.15 1.0]  GraphicEmissiveColor=[0.0 0.0 0.0 1.0]  GraphicShininess=75  GraphicOpacity=0  GeometryShape=Brick  RectangleSize=[1 1]  RectangleSizeUnits=m  BrickDimensions=[L H W]  BrickDimensionUnits=m  CylinderRadius=1  CylinderRadiusUnits=m  CylinderLength=1  CylinderLengthUnits=m  SphereRadius=1  SphereRadiusUnits=m  EllipsoidRadii=[1 1 1]  EllipsoidRadiiUnits=m  ExtrusionCrossSection=[1 1; -1 1; -1 -1; 1 -1]  ExtrusionCrossSectionUnits=m  ExtrusionLength=1  ExtrusionLengthUnits=m  PolygonNumSides=3  PolygonOuterRadius=1  PolygonOuterRadiusUnits=m  ExtGeomFileType=STEP  ExtGeomFileUnits=m  RevolutionCrossSection=[1 1; 1 -1; 2 -1; 2 1]  RevolutionCrossSectionUnits=m  RevolutionExtent=Full  RevolutionAngle=180  RevolutionAngleUnits=deg
  Conn1 : PMIOPort  Port=1  Side=Right
  connections:
  Solid/RConn1 -- Rigid Transform/LConn1
  Rigid Transform/RConn1 -- Conn1/RConn1

== system Jumper_Elastica/Rev-Rot Interface ==
  Ideal Angular Velocity Source : fl_lib/Mechanical/Mechanical Sources/Ideal Angular Velocity Source
  Ideal Torque Sensor : fl_lib/Mechanical/Mechanical Sensors/Ideal Torque Sensor
  w : PMIOPort  Port=1  Side=Right
  R : PMIOPort  Port=2  Side=Right
  t : PMIOPort  Port=3  Side=Left
  C : PMIOPort  Port=4  Side=Left
  connections:
  t/RConn1 -- Ideal Torque Sensor/RConn2
  Ideal Angular Velocity Source/LConn1 -- R/RConn1
  C/RConn1 -- Ideal Torque Sensor/RConn1
  Ideal Torque Sensor/LConn1 -- Ideal Angular Velocity Source/RConn2
  Ideal Angular Velocity Source/RConn1 -- w/RConn1

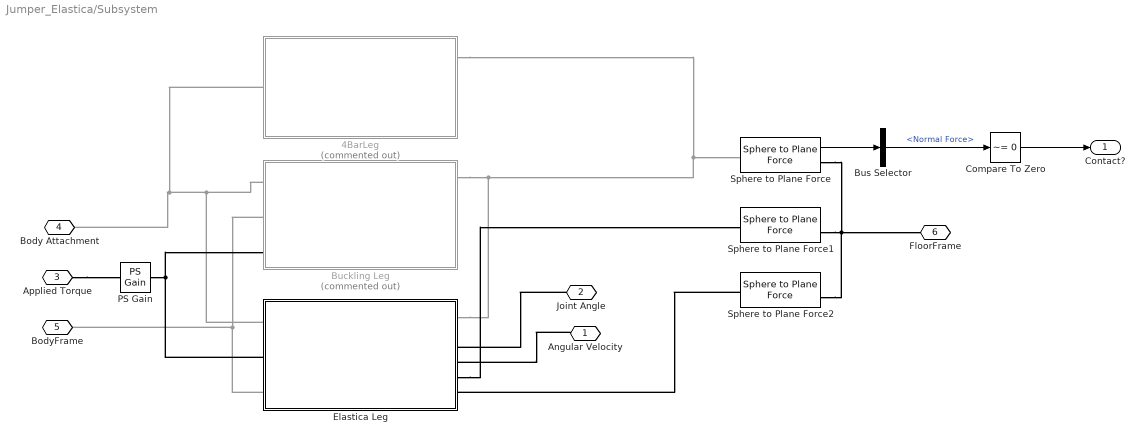
== system Jumper_Elastica/Subsystem ==
  4BarLeg : Subsystem  Commented=on  mask{Knee=Knee, Shin=Shin, FrontThigh=FrontThigh, RearThigh=RearThigh, BaseY=BaseY, BaseX=BaseX, InitialAngle=InitialAngle}
      mask prompts: Knee "Knee (cm)"; Shin "Shin (cm)"; FrontThigh "Front Thigh (cm)"; RearThigh "Rear Thigh  (cm)"; BaseY "BaseY (cm)"; BaseX "BaseX (cm)"; InitialAngle "Initial Angle (deg)"
  Buckling Leg : Subsystem  Commented=on
  Bus Selector : BusSelector  OutputSignals=Normal Force
  Compare To Zero : simulink/Logic and Bit Operations/Compare To Zero  relop=~=  OutDataTypeStr=boolean
  Elastica Leg : Subsystem
  PS Gain : fl_lib/Physical Signals/Functions/PS Gain  gain=1
  Sphere to Plane Force : Contact_Forces_Lib/3D/Sphere to Plane Force  sphere_rad=0.05  plane_lenx=FloorPlaneLength  plane_leny=FloorPlaneWidth  plane_depth=0  force_law=Linear  k_contact=1e4  b_contact=1e3  pen_full_damp_F=1e-4  pen_exponent=1  custom_param_1=1  custom_param_2=1  friction_law=Stick-Slip Continuous  mu_kinetic=JumpingLegDynamicFriction  mu_static=JumpingLegStaticFriction  v_thr=0.001  vis_on=on  vis_opc_en=0  vis_len_plaBz=0.005  vis_clr=[0.9 0.2 0.2]  vis_opc=0.7  mask(Sphere to Plane Force){}
      mask Display: image('D:\Dropbox\MATLAB\SimscapeJumper\SM_Contact_Forces_Lib\SM_Contact_Forces_Lib_R17b_v3p8\Libraries\Images\Sphere_to_Plane_Contact_IMAGE.jpg');
  Sphere to Plane Force1 : Contact_Forces_Lib/3D/Sphere to Plane Force  sphere_rad=0.05  plane_lenx=FloorPlaneLength  plane_leny=FloorPlaneWidth  plane_depth=0  force_law=Linear  k_contact=1e4  b_contact=1e3  pen_full_damp_F=1e-4  pen_exponent=1  custom_param_1=1  custom_param_2=1  friction_law=Stick-Slip Continuous  mu_kinetic=JumpingLegDynamicFriction  mu_static=JumpingLegStaticFriction  v_thr=0.001  vis_on=on  vis_opc_en=0  vis_len_plaBz=0.005  vis_clr=[0.9 0.2 0.2]  vis_opc=0.7  mask(Sphere to Plane Force){}
      mask Display: image('D:\Dropbox\MATLAB\SimscapeJumper\SM_Contact_Forces_Lib\SM_Contact_Forces_Lib_R17b_v3p8\Libraries\Images\Sphere_to_Plane_Contact_IMAGE.jpg');
  Sphere to Plane Force2 : Contact_Forces_Lib/3D/Sphere to Plane Force  sphere_rad=0.05  plane_lenx=FloorPlaneLength  plane_leny=FloorPlaneWidth  plane_depth=0  force_law=Linear  k_contact=1e4  b_contact=1e3  pen_full_damp_F=1e-4  pen_exponent=1  custom_param_1=1  custom_param_2=1  friction_law=Stick-Slip Continuous  mu_kinetic=JumpingLegDynamicFriction  mu_static=JumpingLegStaticFriction  v_thr=0.001  vis_on=on  vis_opc_en=0  vis_len_plaBz=0.005  vis_clr=[0.9 0.2 0.2]  vis_opc=0.7  mask(Sphere to Plane Force){}
      mask Display: image('D:\Dropbox\MATLAB\SimscapeJumper\SM_Contact_Forces_Lib\SM_Contact_Forces_Lib_R17b_v3p8\Libraries\Images\Sphere_to_Plane_Contact_IMAGE.jpg');
  Angular Velocity : PMIOPort  Port=1  Side=Right
  Joint Angle : PMIOPort  Port=2  Side=Right
  Applied Torque : PMIOPort  Port=3  Side=Left
  Body Attachment : PMIOPort  Port=4  Side=Left
  BodyFrame : PMIOPort  Port=5  Side=Left
  FloorFrame : PMIOPort  Port=6  Side=Right
  Contact? : Outport
  wires:
  Sphere to Plane Force/1 -> Bus Selector/1
  Bus Selector/1 -> Compare To Zero/1  "<Normal Force>"
  Compare To Zero/1 -> Contact?/1
  connections:
  Sphere to Plane Force/RConn1 -- Sphere to Plane Force2/RConn1 -- FloorFrame/RConn1 -- Sphere to Plane Force1/RConn1
  Buckling Leg/LConn1 -- Elastica Leg/LConn1 -- 4BarLeg/LConn2 -- Body Attachment/RConn1
  Buckling Leg/LConn2 -- BodyFrame/RConn1 -- Elastica Leg/LConn3
  4BarLeg/RConn1 -- Elastica Leg/RConn1 -- Buckling Leg/RConn1 -- Sphere to Plane Force/LConn1
  Elastica Leg/RConn5 -- Sphere to Plane Force1/LConn1
  Sphere to Plane Force2/LConn1 -- Elastica Leg/RConn6
  Applied Torque/RConn1 -- PS Gain/LConn1
  PS Gain/RConn1 -- Elastica Leg/LConn2 -- Buckling Leg/LConn3
  Joint Angle/RConn1 -- Elastica Leg/RConn3
  Angular Velocity/RConn1 -- Elastica Leg/RConn4

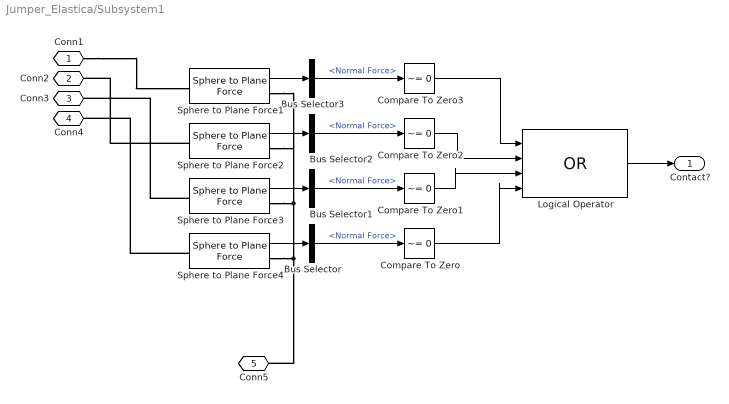
== system Jumper_Elastica/Subsystem1 ==
  Bus Selector{,1..3} (4 alike) : BusSelector  OutputSignals=Normal Force
  Compare To Zero{,1..3} (4 alike) : simulink/Logic and Bit Operations/Compare To Zero  relop=~=  OutDataTypeStr=boolean
  Logical Operator : Logic  Operator=OR  Inputs=4  IconShape=distinctive  AllPortsSameDT=off  OutDataTypeStr=boolean
  Sphere to Plane Force{1..4} (4 alike) : Contact_Forces_Lib/3D/Sphere to Plane Force  sphere_rad=0.05  plane_lenx=FloorPlaneLength  plane_leny=FloorPlaneWidth  plane_depth=0  force_law=Linear  k_contact=1e4  b_contact=1e3  pen_full_damp_F=1e-4  pen_exponent=1  custom_param_1=1  custom_param_2=1  friction_law=Stick-Slip Continuous  mu_kinetic=LandingLegDynamicFriction  mu_static=LandingLegStaticFriction  v_thr=0.001  vis_on=on  vis_opc_en=0  vis_len_plaBz=0.005  vis_clr=[0.9 0.2 0.2]  vis_opc=0.7  mask(Sphere to Plane Force){}
      mask Display: image('D:\Dropbox\MATLAB\SimscapeJumper\SM_Contact_Forces_Lib\SM_Contact_Forces_Lib_R17b_v3p8\Libraries\Images\Sphere_to_Plane_Contact_IMAGE.jpg');
  Conn1 : PMIOPort  Port=1  Side=Left
  Conn2 : PMIOPort  Port=2  Side=Left
  Conn3 : PMIOPort  Port=3  Side=Left
  Conn4 : PMIOPort  Port=4  Side=Left
  Conn5 : PMIOPort  Port=5  Side=Left
  Contact? : Outport
  wires:
  Sphere to Plane Force4/1 -> Bus Selector/1
  Bus Selector/1 -> Compare To Zero/1  "<Normal Force>"
  Sphere to Plane Force3/1 -> Bus Selector1/1
  Bus Selector1/1 -> Compare To Zero1/1  "<Normal Force>"
  Compare To Zero1/1 -> Logical Operator/3
  Sphere to Plane Force2/1 -> Bus Selector2/1
  Bus Selector2/1 -> Compare To Zero2/1  "<Normal Force>"
  Compare To Zero2/1 -> Logical Operator/2
  Sphere to Plane Force1/1 -> Bus Selector3/1
  Bus Selector3/1 -> Compare To Zero3/1  "<Normal Force>"
  Compare To Zero3/1 -> Logical Operator/1
  Compare To Zero/1 -> Logical Operator/4
  Logical Operator/1 -> Contact?/1
  connections:
  Sphere to Plane Force4/RConn1 -- Conn5/RConn1 -- Sphere to Plane Force3/RConn1 -- Sphere to Plane Force2/RConn1 -- Sphere to Plane Force1/RConn1
  Conn1/RConn1 -- Sphere to Plane Force1/LConn1
  Sphere to Plane Force2/LConn1 -- Conn2/RConn1
  Sphere to Plane Force3/LConn1 -- Conn3/RConn1
  Sphere to Plane Force4/LConn1 -- Conn4/RConn1

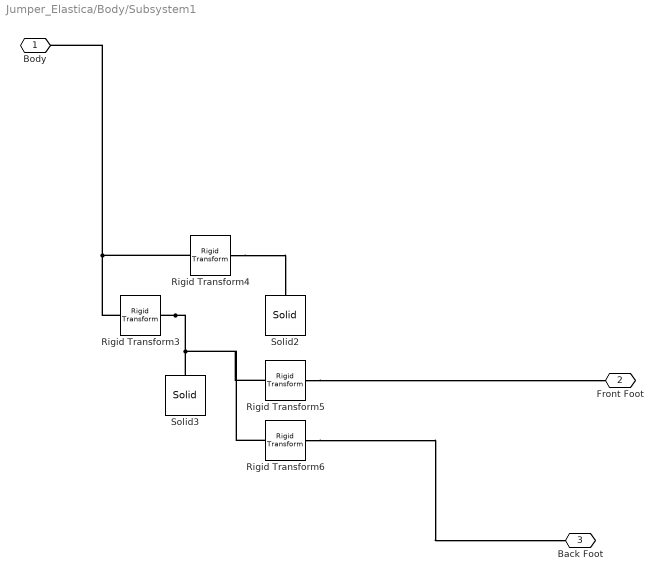
== system Jumper_Elastica/Body/Subsystem1 ==
  Rigid Transform3 : sm_lib/Frames and Transforms/Rigid Transform  TranslationMethod=Cartesian  TranslationStandardOffset=L/4  TranslationLengthUnit=m  TranslationStandardAxis=+Y  TranslationCartesianOffset=[0 -LegH 0]  TranslationROffset=0  TranslationROffsetUnits=m  TranslationZOffset=0  TranslationZOffsetUnits=m  TranslationThetaOffset=0  TranslationThetaOffsetUnits=deg  RotationMethod=AlignedAxes  RotationAngleUnits=deg  RotationStandardAxis=+X  RotationAngle=90  RotationArbitraryAxis=[0 0 1]  FollAlignAxisA=+Z  BaseAlignAxisA=+X  FollAlignAxisB=+Y  BaseAlignAxisB=+Z  RotationSequenceAxes=BaseAxes  RotationSequence=XYX  RotationSequenceAngles=[0 0 0]  RotationSequenceAnglesUnits=deg  RotationMatrix=[1 0 0; 0 1 0; 0 0 1]
  Rigid Transform4 : sm_lib/Frames and Transforms/Rigid Transform  TranslationMethod=Cartesian  TranslationStandardOffset=L/4  TranslationLengthUnit=m  TranslationStandardAxis=+Y  TranslationCartesianOffset=[0 -LegH/2 0]  TranslationROffset=0  TranslationROffsetUnits=m  TranslationZOffset=0  TranslationZOffsetUnits=m  TranslationThetaOffset=0  TranslationThetaOffsetUnits=deg  RotationMethod=AlignedAxes  RotationAngleUnits=deg  RotationStandardAxis=+X  RotationAngle=90  RotationArbitraryAxis=[0 0 1]  FollAlignAxisA=+Z  BaseAlignAxisA=-Y  FollAlignAxisB=+Y  BaseAlignAxisB=+X  RotationSequenceAxes=BaseAxes  RotationSequence=XYX  RotationSequenceAngles=[0 0 0]  RotationSequenceAnglesUnits=deg  RotationMatrix=[1 0 0; 0 1 0; 0 0 1]
  Rigid Transform5 : sm_lib/Frames and Transforms/Rigid Transform  TranslationMethod=StandardAxis  TranslationStandardOffset=LegL/2  TranslationLengthUnit=m  TranslationStandardAxis=+Z  TranslationCartesianOffset=[0 -LegH 0]  TranslationROffset=0  TranslationROffsetUnits=m  TranslationZOffset=0  TranslationZOffsetUnits=m  TranslationThetaOffset=0  TranslationThetaOffsetUnits=deg  RotationMethod=None  RotationAngleUnits=deg  RotationStandardAxis=+X  RotationAngle=90  RotationArbitraryAxis=[0 0 1]  FollAlignAxisA=+Z  BaseAlignAxisA=+X  FollAlignAxisB=+Y  BaseAlignAxisB=+Z  RotationSequenceAxes=BaseAxes  RotationSequence=XYX  RotationSequenceAngles=[0 0 0]  RotationSequenceAnglesUnits=deg  RotationMatrix=[1 0 0; 0 1 0; 0 0 1]
  Rigid Transform6 : sm_lib/Frames and Transforms/Rigid Transform  TranslationMethod=StandardAxis  TranslationStandardOffset=LegL/2  TranslationLengthUnit=m  TranslationStandardAxis=-Z  TranslationCartesianOffset=[0 -LegH 0]  TranslationROffset=0  TranslationROffsetUnits=m  TranslationZOffset=0  TranslationZOffsetUnits=m  TranslationThetaOffset=0  TranslationThetaOffsetUnits=deg  RotationMethod=None  RotationAngleUnits=deg  RotationStandardAxis=+X  RotationAngle=90  RotationArbitraryAxis=[0 0 1]  FollAlignAxisA=+Z  BaseAlignAxisA=+X  FollAlignAxisB=+Y  BaseAlignAxisB=+Z  RotationSequenceAxes=BaseAxes  RotationSequence=XYX  RotationSequenceAngles=[0 0 0]  RotationSequenceAnglesUnits=deg  RotationMatrix=[1 0 0; 0 1 0; 0 0 1]
  Solid2 : sm_lib/Body Elements/Solid  InertiaType=CalculateFromGeometry  Mass=LegM/4  MassUnits=kg  CenterOfMass=[0 0 0]  CenterOfMassUnits=m  MomentsOfInertia=[1 1 1]  MomentsOfInertiaUnits=kg*m^2  ProductsOfInertia=[1 1 1]  ProductsOfInertiaUnits=kg*m^2  DensityBased=off  Density=1000  DensityUnits=kg/m^3  DoExposeReferenceFrame=on  SerializedFrames=<Frames/>  GraphicType=FromGeometry  MarkerShape=Sphere  MarkerSize=10  GraphicVisPropType=SimpleVisualProperties  GraphicDiffuseColor=rgb  GraphicSpecularColor=[0.5 0.5 0.5 1.0]  GraphicAmbientColor=[0.15 0.15 0.15 1.0]  GraphicEmissiveColor=[0.0 0.0 0.0 1.0]  GraphicShininess=75  GraphicOpacity=1.0  GeometryShape=Cylinder  RectangleSize=[1 1]  RectangleSizeUnits=m  BrickDimensions=[L H W]  BrickDimensionUnits=m  CylinderRadius=0.01  CylinderRadiusUnits=m  CylinderLength=LegH  CylinderLengthUnits=m  SphereRadius=1  SphereRadiusUnits=m  EllipsoidRadii=[1 1 1]  EllipsoidRadiiUnits=m  ExtrusionCrossSection=[1 1; -1 1; -1 -1; 1 -1]  ExtrusionCrossSectionUnits=m  ExtrusionLength=1  ExtrusionLengthUnits=m  PolygonNumSides=3  PolygonOuterRadius=1  PolygonOuterRadiusUnits=m  ExtGeomFileType=STEP  ExtGeomFileUnits=m  RevolutionCrossSection=[1 1; 1 -1; 2 -1; 2 1]  RevolutionCrossSectionUnits=m  RevolutionExtent=Full  RevolutionAngle=180  RevolutionAngleUnits=deg
  Solid3 : sm_lib/Body Elements/Solid  InertiaType=CalculateFromGeometry  Mass=LegM/4  MassUnits=kg  CenterOfMass=[0 0 0]  CenterOfMassUnits=m  MomentsOfInertia=[1 1 1]  MomentsOfInertiaUnits=kg*m^2  ProductsOfInertia=[1 1 1]  ProductsOfInertiaUnits=kg*m^2  DensityBased=off  Density=1000  DensityUnits=kg/m^3  DoExposeReferenceFrame=on  SerializedFrames=<Frames/>  GraphicType=FromGeometry  MarkerShape=Sphere  MarkerSize=10  GraphicVisPropType=SimpleVisualProperties  GraphicDiffuseColor=rgb  GraphicSpecularColor=[0.5 0.5 0.5 1.0]  GraphicAmbientColor=[0.15 0.15 0.15 1.0]  GraphicEmissiveColor=[0.0 0.0 0.0 1.0]  GraphicShininess=75  GraphicOpacity=1.0  GeometryShape=Cylinder  RectangleSize=[1 1]  RectangleSizeUnits=m  BrickDimensions=[L H W]  BrickDimensionUnits=m  CylinderRadius=0.01  CylinderRadiusUnits=m  CylinderLength=LegL  CylinderLengthUnits=m  SphereRadius=1  SphereRadiusUnits=m  EllipsoidRadii=[1 1 1]  EllipsoidRadiiUnits=m  ExtrusionCrossSection=[1 1; -1 1; -1 -1; 1 -1]  ExtrusionCrossSectionUnits=m  ExtrusionLength=1  ExtrusionLengthUnits=m  PolygonNumSides=3  PolygonOuterRadius=1  PolygonOuterRadiusUnits=m  ExtGeomFileType=STEP  ExtGeomFileUnits=m  RevolutionCrossSection=[1 1; 1 -1; 2 -1; 2 1]  RevolutionCrossSectionUnits=m  RevolutionExtent=Full  RevolutionAngle=180  RevolutionAngleUnits=deg
  Body : PMIOPort  Port=1  Side=Left
  Front Foot : PMIOPort  Port=2  Side=Right
  Back Foot : PMIOPort  Port=3  Side=Right
  connections:
  Rigid Transform3/RConn1 -- Solid3/RConn1 -- Rigid Transform5/LConn1 -- Rigid Transform6/LConn1
  Rigid Transform6/RConn1 -- Back Foot/RConn1
  Rigid Transform5/RConn1 -- Front Foot/RConn1
  Rigid Transform3/LConn1 -- Rigid Transform4/LConn1 -- Body/RConn1
  Rigid Transform4/RConn1 -- Solid2/RConn1
